simulink model "generateData"  (R2022a)
settings: Solver=FixedStepAuto  StartTime=0.0  StopTime=tend  FixedStep=0.01  RelTol=1e-3
undefined symbols (not defined in the file): center, epsilon, mergepose, pwo_init, scale, v
libraries: simlib_vpc_basic x4, simlib_vpc_coremath x2
settings Model: Creator=marco  LastModifiedBy=marco
settings DebuggingCC: AlgebraicLoopMsg=none  ArtificialAlgebraicLoopMsg=none  UnconnectedInputMsg=warning  UnconnectedOutputMsg=warning  UnconnectedLineMsg=warning
settings RTWCC: DLArmComputeVersion=19.05

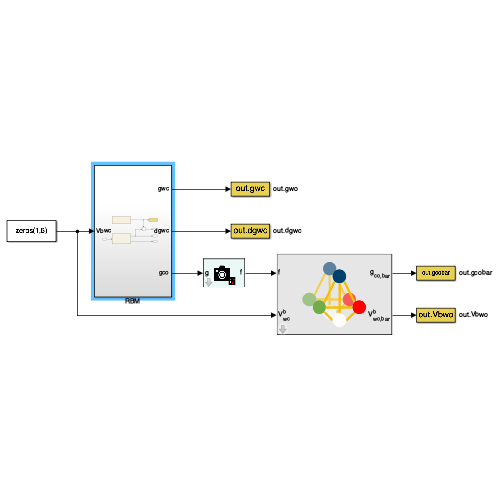
[thumbnail: Simulink's stored preview of the top-level diagram]
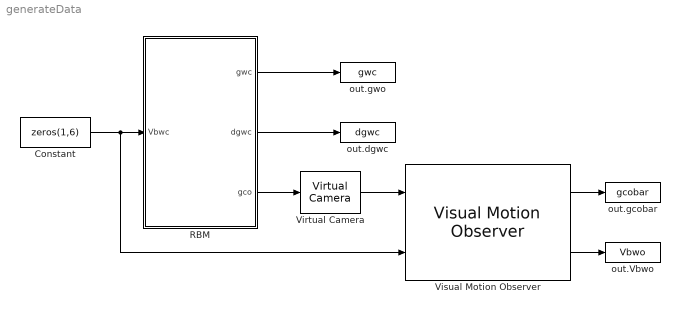
== system generateData ==
  Constant : Constant  Value=zeros(1,6)
  RBM : Subsystem
  Virtual Camera : simlib_vpc_basic/Virtual Camera  camtype=Pinhole  po=fp  lambda=lambda
      settings: SourceProductName=VPC Library
  Visual Motion Observer : simlib_vpc_basic/Visual Motion Observer  show_ee=off  show_gee=off  show_Vbwo=on  show_dgcobar=off  show_ue_aux=off  gcobar0=mergepose(eye(3),[0 1 0])  projection=on  Ke_source=internal  Ke=Ke  camtype=Pinhole  fo=fp  lambda=lambda
      settings: SourceProductName=VPC Library
  out.Vbwo : ToWorkspace  VariableName=Vbwo  SaveFormat=Structure With Time  SampleTime=-1
  out.dgwc : ToWorkspace  VariableName=dgwc  SaveFormat=Structure With Time  SampleTime=-1
  out.gcobar : ToWorkspace  VariableName=gcobar  SaveFormat=Structure With Time  SampleTime=-1
  out.gwo : ToWorkspace  VariableName=gwc  SaveFormat=Structure With Time  SampleTime=-1
  wires:
  Virtual Camera/1 -> Visual Motion Observer/1
  Constant/1 -> Visual Motion Observer/2, RBM/1(Vbwc)
  Visual Motion Observer/1 -> out.gcobar/1
  RBM/3(gco) -> Virtual Camera/1
  RBM/1(gwc) -> out.gwo/1
  RBM/2(dgwc) -> out.dgwc/1
  Visual Motion Observer/2 -> out.Vbwo/1

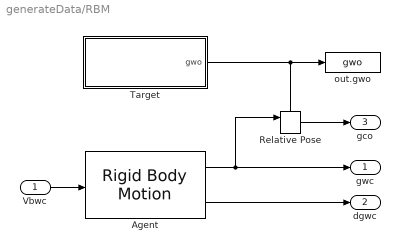
== system generateData/RBM ==
  Vbwc : Inport
  Agent : simlib_vpc_basic/Rigid Body Motion  rbmtype=agent  agentnumber=1  projection=on  show_dg=on  g0=gwc_init
      settings: SourceProductName=VPC Library
  Relative Pose : simlib_vpc_coremath/Relative Pose
      settings: SourceProductName=VPC Library
  Target : Subsystem
      mask Display:
      | % Glitch in Matlab: If you define a line whose starting point and end point
      | % is equal, then the entire mask block is plotted in bold
      | plot([0,0],[0,0])
      | 
      | % Draw Box
      | plot([0,1,1,0,0],[0,0,1,1,0])
      | 
      | % Write label
      | disp('Target','texmode','on')
      | 
      | % Image
      | p=get_param(gcb,'Position');
      | size = min(p(3:4)-p(1:2));
      | blkscale = abs((p(3)-p(1)) / (p(4)-p(2)));
      | if abs((p(3)-p(1))) > abs((p(4)-p(2))) % block is horizontal
      |     scale = .5*[1/blkscale .6];
      | else % block is vertical
      |     scale = .5*[1 .6*blkscale];
      | end
      | pos = [1-scale(1) 0.1]/2;
      | image('ico_target.png',[pos scale],'off')
      | 
      | % Label ports
      | port_label('output',1,['g_{wo}'],'texmode','on')
  out.gwo : ToWorkspace  VariableName=gwo  SaveFormat=Structure With Time  SampleTime=-1
  gwc : Outport
  dgwc : Outport  Port=2
  gco : Outport  Port=3
  wires:
  Vbwc/1 -> Agent/1
  Agent/1 -> Relative Pose/1, gwc/1
  Agent/2 -> dgwc/1
  Relative Pose/1 -> gco/1
  Target/1(gwo) -> Relative Pose/2, out.gwo/1

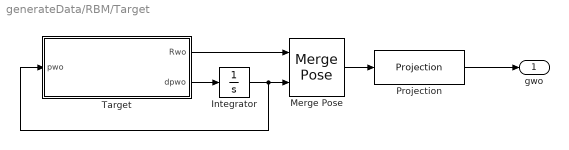
== system generateData/RBM/Target ==
  Integrator : Integrator  InitialCondition=pwo_init  ContinuousStateAttributes='pose'
  Merge Pose : simlib_vpc_coremath/Merge Pose
      settings: SourceProductName=VPC Library
  Projection : simlib_vpc_basic/Projection  projectiontype=averaging  inputtype=pose
      settings: SourceProductName=VPC Library
  Target : MATLAB Function  TreatAsAtomicUnit=on
  gwo : Outport
  wires:
  Merge Pose/1 -> Projection/1
  Projection/1 -> gwo/1
  Integrator/1 -> Target/1(pwo), Merge Pose/2
  Target/2(dpwo) -> Integrator/1
  Target/1(Rwo) -> Merge Pose/1

== matlab function generateData/RBM/Target/Target ==
  data: pwo input; v parameter; Rwo output; dpwo output; epsilon parameter; scale parameter; center parameter
function [Rwo, dpwo] = target_trajectory(pwo, v, epsilon, scale, center) %#codegen
% Target Movement
%
% Editor:
%   OMAINSKA Marco - Doctoral Student, Cybernetics
%       <marcoomainska@g.ecc.u-tokyo.ac.jp>
% Review:
%   YAMAUCHI Junya - Assistant Professor
%       <junya_yamauchi@ipc.i.u-tokyo.ac.jp>
%
% Property of: Fujita-Yamauchi Lab, University of Tokyo, 2023
% Website: https://www.scl.ipc.i.u-tokyo.ac.jp
%
%------------- BEGIN CODE --------------

% Get velocity
% Vb = vanderpol(pwo,v,epsilon,center,scale);
Vb = quartic(pwo,v,epsilon,center,scale);
dpwo = Vb(1:3);

% set heading angle
zangle = rad2deg(atan2(dpwo(2),dpwo(1)) - pi/2);
alpha = rad2deg(asin( dpwo(3)/norm(dpwo,2) ));
Rwo = rotz(zangle)*rotx(alpha);

%------------- END CODE --------------
end
